simulink model "ComputeCoherence"  (R2016b)
settings: Solver=FixedStepDiscrete  StartTime=0.0  StopTime=Inf  FixedStep=sCoreParams.core.stepPeriod  RelTol=1e-3  EnableMultiTasking=on
undefined symbols (not defined in the file): Low, sCoreParams
libraries: dspswit3 x1
settings Model: DataTypeOverride=Double  MinMaxOverflowLogging=ForceOff  Creator=rzelmann  LastModifiedBy=Rina
settings SolverCC: EnableConcurrentExecution=on  ConcurrentTasks=on  AutoInsertRateTranBlk=on
settings DataIOCC: SaveFormat=StructureWithTime
settings OptimizationCC: BlockReduction=off  DefaultParameterBehavior=Inlined  OptimizeBlockIOStorage=off  BufferReuse=off  GlobalBufferReuse=off  ExpressionFolding=off  LocalBlockOutputs=off  EfficientFloat2IntCast=on  LifeSpan=inf
settings DebuggingCC: SFUnexpectedBacktrackingDiag=warning  SFNoUnconditionalDefaultTransitionDiag=warning  SFExecutionAtInitializationDiag=none
settings HardwareCC: ProdBitPerPointer=32  ProdBitPerSizeT=32  ProdBitPerPtrDiffT=32  ProdLargestAtomicFloat=None  ProdWordSize=32  ProdLongLongMode=on  ProdHWDeviceType=Generic->32-bit x86 compatible
settings ModelReferenceCC: ModelReferenceNumInstancesAllowed=Single  ModelReferencePassRootInputsByReference=off
settings RTWCC: SystemTargetFile=slrt.tlc  TemplateMakefile=slrt_default_tmf  Description=Simulink Real-Time  RTWCompilerOptimization=on
settings TargetCC: CodeReplacementLibrary=XPC_BLAS  ParMdlRefBuildCompliant=on  ConcurrentExecutionCompliant=on  GeneratePreprocessorConditionals=Use local settings  MatFileLogging=on  MATLABClassNameForMDSCustomization=xpcAperiodicCustomization
settings ConfigComp: CovMetricSettings=dw  CovHtmlReporting=on  CovSaveCumulativeToWorkspaceVar=on  CovSaveSingleToWorkspaceVar=on  CovExternalEMLEnable=off

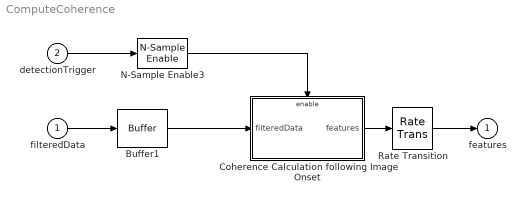
== system ComputeCoherence ==
  filteredData : Inport  PortDimensions=[sCoreParams.core.samplesPerStep sCoreParams.decoders.txDetector.nFilteredChannels]  SampleTime=sCoreParams.core.stepPeriod
  detectionTrigger : Inport  Port=2  OutDataTypeStr=boolean  PortDimensions=1  SampleTime=sCoreParams.core.stepPeriod
  Buffer1 : Buffer  N=sCoreParams.Features.Coherence.WindowDurationSamples  V=sCoreParams.Features.Coherence.WindowDurationSamples-sCoreParams.core.samplesPerStep  TreatMby1Signals=One channel
  "Coherence Calculation following Image Onset " : Subsystem
  N-Sample Enable3 : dspswit3/N-Sample Enable  N=sCoreParams.decoders.txDetector.detectionDurationSteps  ActiveLevel=Low (0)  reset=on  TriggerType=Rising edge  Ts=1  DataType=Logical
  Rate Transition : RateTransition
  features : Outport  SampleTime=sCoreParams.core.stepPeriod
  wires:
  filteredData/1 -> Buffer1/1
  Rate Transition/1 -> features/1
  detectionTrigger/1 -> N-Sample Enable3/1
  Buffer1/1 -> "Coherence Calculation following Image Onset "/1(filteredData)
  "Coherence Calculation following Image Onset "/1(features) -> Rate Transition/1
  N-Sample Enable3/1 -> "Coherence Calculation following Image Onset "/Enable

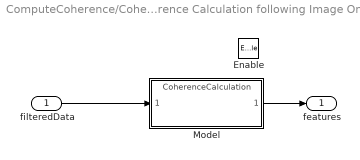
== system ComputeCoherence/Coherence Calculation following Image Onset  ==
  filteredData : Inport
  Enable : EnablePort
  Model : ModelReference  ModelNameDialog=CoherenceCalculation.slx  SimulationMode=Normal  ModelReferenceVersion=1.512
  features : Outport
  wires:
  filteredData/1 -> Model/1
  Model/1 -> features/1
